simulink model "ld3_floting_point"  (R2017b)
settings: Solver=VariableStepAuto  StartTime=0.0  StopTime=0.01  RelTol=1e-3
settings Model: SimulationMode=accelerator  Creator=Imants  LastModifiedBy=Imants

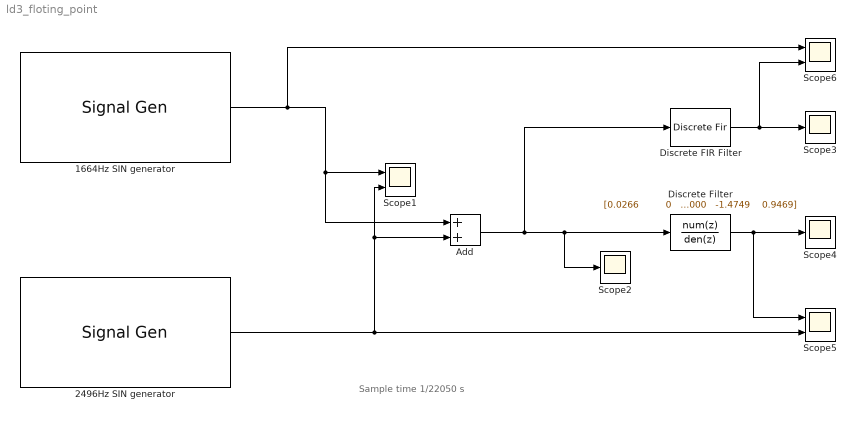
== system ld3_floting_point ==
  note: Sample time 1/22050 s
  1664Hz SIN generator : SignalGenerator  Frequency=1664
  2496Hz SIN generator : SignalGenerator  Frequency=2496
  Add : Sum
  Discrete FIR Filter : DiscreteFir  Coefficients="[-0.0073   -0.0071   -0.0059   -0.0024    0.0040    0.0133    0.0231    0.0301    0.0302    0.0207    0.0014   -0.0242   -0.0498 -0.0677   -0.0713   -0.0571   -0.0269    0.0129    0.0525    0.0814    0.0921    0.0814    0.0525    0.0129   -0.0269   -0.0571 -0.0713   -0.0677   -0.0498   -0.0242    0.0014    0.0207    0.0302    0.0301    0.0231    0.0133    0.0040   -0.0024   -0.0059 -0.0071   -0.0073]"
  Discrete Filter : DiscreteFilter  Numerator="[0.0266         0   -0.0266]"  Denominator="[1.0000   -1.4749    0.9469]"  InputProcessing=Columns as channels (frame based)
  Scope1 : Scope  NumInputPorts=2
  Scope2 : Scope
  Scope3 : Scope
  Scope4 : Scope
  Scope5 : Scope  NumInputPorts=2
  Scope6 : Scope  NumInputPorts=2
  wires:
  Add/1 -> Discrete FIR Filter/1, Scope2/1, Discrete Filter/1
  1664Hz SIN generator/1 -> Scope6/1, Scope1/1, Add/1
  2496Hz SIN generator/1 -> Scope1/2, Add/2, Scope5/2
  Discrete Filter/1 -> Scope5/1, Scope4/1
  Discrete FIR Filter/1 -> Scope6/2, Scope3/1
